simulink model "test_notch"  (R2022b)
settings: Solver=VariableStepAuto  StartTime=0.0  StopTime=10  RelTol=1e-3
undefined symbols (not defined in the file or in its folder): notch
libraries: dspsrcs4 x1
settings Model: Creator=peter  LastModifiedBy=peter

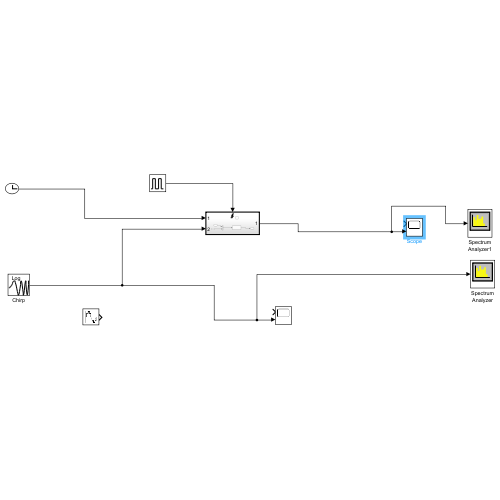
[thumbnail: Simulink's stored preview of the top-level diagram]
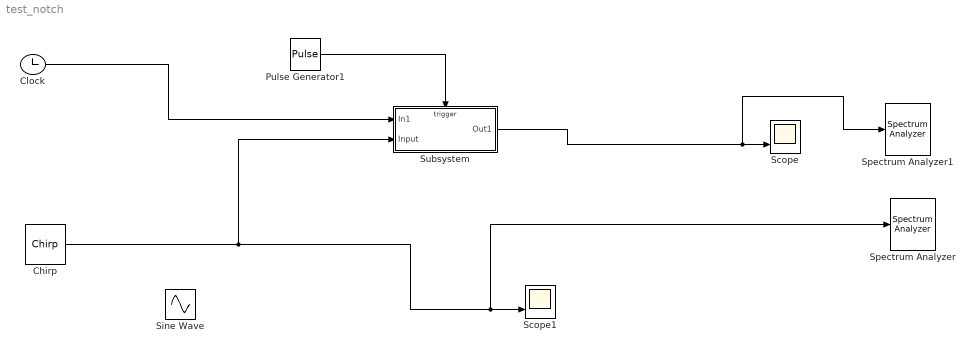
== system test_notch ==
  Chirp : dspsrcs4/Chirp  sweep=Logarithmic  mode=Unidirectional  f0=0.1  f1=4000  t1=10  Tsweep=20  phase=0  Ts=0.001  spf=1  datatype=Double  OutputFrames=off
  Clock : Clock
      settings: Decimation=100000
  Pulse Generator1 : DiscretePulseGenerator  PulseType=Time based  Period=0.001  PulseWidth=50
  Scope : Scope  NumInputPorts=2
  Scope1 : Scope  NumInputPorts=2
  Sine Wave : Sin  Amplitude=10  SampleTime=0.001
  Spectrum Analyzer : SpectrumAnalyzer
  Spectrum Analyzer1 : SpectrumAnalyzer
  Subsystem : Subsystem
  wires:
  Subsystem/1(Out1) -> Spectrum Analyzer1/1, Scope/2
  Pulse Generator1/1 -> Subsystem/Trigger
  Clock/1 -> Subsystem/1(In1)
  Chirp/1 -> Subsystem/2(Input), Spectrum Analyzer/1, Scope1/2

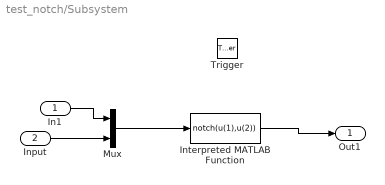
== system test_notch/Subsystem ==
  In1 : Inport
  Input : Inport  Port=2
  Trigger : TriggerPort  VariantControl=(inherit)  PortDimensions=1
  Interpreted MATLAB Function : MATLABFcn  MATLABFcn=notch(u(1),u(2))
  Mux : Mux  Inputs=2
  Out1 : Outport
  wires:
  Mux/1 -> Interpreted MATLAB Function/1
  In1/1 -> Mux/1
  Interpreted MATLAB Function/1 -> Out1/1
  Input/1 -> Mux/2
